simulink model "system_model_user_friendly"  (R2013a)
settings: Solver=ode15s  StartTime=0.0  StopTime=20  FixedStep=.00001  MaxStep=0.001  RelTol=1e-3
values from neighbouring files (symbols this model uses):
  Ga = 3    [a2_data_input_examsim1.m]    (also in a2_data_input_examsim2.m = 1; a2_data_input_hw3.m = 0.095; a2_data_input_mdcs_h5_v1_stud_p1.m = 0.095; a2_data_input_mdcs_h5_v1_stud_p4.m = 0.006)
  Gf = Gr/(Kd*Gs)    [a3_process_input.m]
  Gs = 1    [a2_data_input_examsim1.m]    (also in a2_data_input_examsim2.m = 5; a2_data_input_hw3.m; a2_data_input_mdcs_h5_v1_stud_p1.m; a2_data_input_mdcs_h5_v1_stud_p4.m)
  Kd = 2    [a2_data_input_examsim1.m]    (also in a2_data_input_examsim2.m = 1; a2_data_input_hw3.m = 1; a2_data_input_mdcs_h5_v1_stud_p1.m = 1; a2_data_input_mdcs_h5_v1_stud_p4.m = 1)
undefined symbols (not defined in the file or in its folder): da, dp, ds, r
libraries: cstblocks x2
settings Model: Creator=s177063  LastModifiedBy=Vittorio
settings DataIOCC: ExternalInput=[t,u]  LimitDataPoints=off  SaveOutput=off
settings OptimizationCC: ExpressionDepthLimit=2147483647
settings DebuggingCC: UnderspecifiedInitializationDetection=Simplified
settings GRTTargetCC: CombineOutputUpdateFcns=off  GRTInterface=on

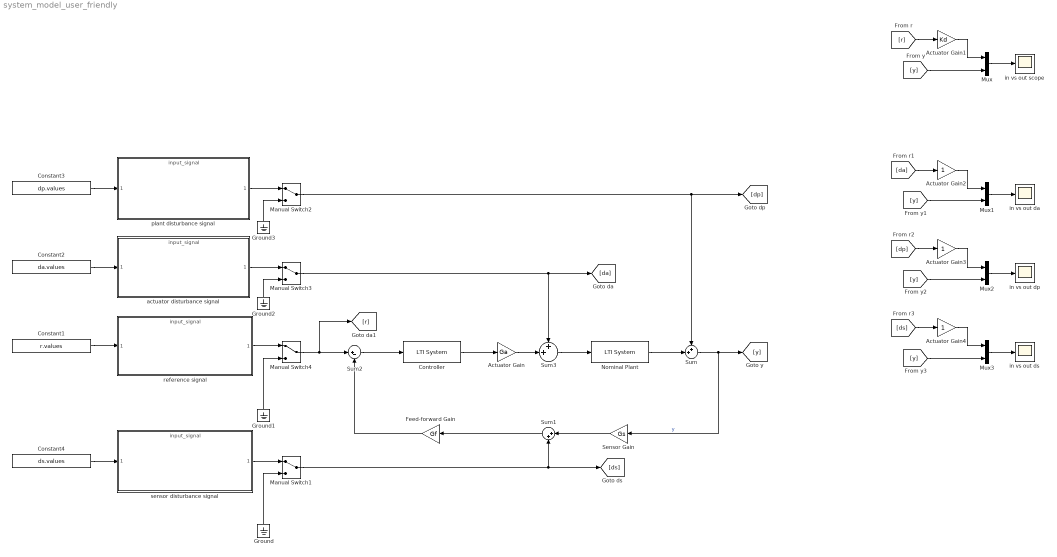
== system system_model_user_friendly ==
  Actuator Gain : Gain  Gain=Ga
  Actuator Gain1 : Gain  Gain=Kd
  Actuator Gain2 : Gain
  Actuator Gain3 : Gain
  Actuator Gain4 : Gain
  Constant1 : Constant  Value=r.values  OutDataTypeStr=Bus: slBus1
  Constant2 : Constant  Value=da.values  OutDataTypeStr=Bus: slBus1
  Constant3 : Constant  Value=dp.values  OutDataTypeStr=Bus: slBus1
  Constant4 : Constant  Value=ds.values  OutDataTypeStr=Bus: slBus1
  Controller : cstblocks/LTI System  sys=Gc.mod.value  IC=[]
  Feed-forward Gain : Gain  Gain=Gf
  Ground{,1..3} (4 alike) : Ground
  Manual Switch{1..4} (4 alike) : ManualSwitch
  Mux{,1..3} (4 alike) : Mux  Inputs=2
  Nominal Plant : cstblocks/LTI System  sys=Gp.nominal.tf  IC=[]
  Sensor Gain : Gain  Gain=Gs
  Sum : Sum  Inputs=++|
  Sum1 : Sum  Inputs=|++
  Sum2 : Sum  Inputs=|+-
  Sum3 : Sum  Inputs=++|
  actuator disturbance signal : ModelReference  ModelNameDialog=input_signal  ModelReferenceVersion=1.24  CopyOfModelName=input_signal  DefaultDataLogging=off
  in vs out da : Scope
      settings: TimeRange=0.5  YMin=0.00425  YMax=0.0085  SampleInput=on
  in vs out dp : Scope
      settings: TimeRange=0.5  YMin=7.45  YMax=8.3  SaveName=ScopeData2  SampleInput=on
  in vs out ds : Scope
      settings: TimeRange=0.5  YMin=-0.0012  YMax=0.0012  SaveName=ScopeData3  SampleInput=on
  in vs out scope : Scope
      settings: TimeRange=0.5  YMin=7.45  YMax=8.3  SampleInput=on
  plant disturbance signal : ModelReference  ModelNameDialog=input_signal  ModelReferenceVersion=1.24  CopyOfModelName=input_signal  DefaultDataLogging=off
  reference signal : ModelReference  ModelNameDialog=input_signal  ModelReferenceVersion=1.24  CopyOfModelName=input_signal  DefaultDataLogging=off
  sensor disturbance signal : ModelReference  ModelNameDialog=input_signal  ModelReferenceVersion=1.24  CopyOfModelName=input_signal  DefaultDataLogging=off
  wires:
  Sum/1 -> Sensor Gain/1, [y]  "y"
  Controller/1 -> Actuator Gain/1
  Sum3/1 -> Nominal Plant/1
  Sum2/1 -> Controller/1
  Sensor Gain/1 -> Sum1/1
  Sum1/1 -> Feed-forward Gain/1
  Feed-forward Gain/1 -> Sum2/2
  Actuator Gain/1 -> Sum3/2
  Nominal Plant/1 -> Sum/2
  Mux/1 -> in vs out scope/1
  [r] -> Actuator Gain1/1
  Actuator Gain1/1 -> Mux/1
  [y] -> Mux/2
  Constant1/1 -> reference signal/1
  Constant2/1 -> actuator disturbance signal/1
  Constant3/1 -> plant disturbance signal/1
  Constant4/1 -> sensor disturbance signal/1
  plant disturbance signal/1 -> Manual Switch2/1
  Manual Switch2/1 -> Sum/1, [dp]
  actuator disturbance signal/1 -> Manual Switch3/1
  reference signal/1 -> Manual Switch4/1
  Manual Switch4/1 -> [r], Sum2/1
  sensor disturbance signal/1 -> Manual Switch1/1
  Manual Switch1/1 -> Sum1/2, [ds]
  Ground/1 -> Manual Switch1/2
  Ground1/1 -> Manual Switch4/2
  Ground2/1 -> Manual Switch3/2
  Ground3/1 -> Manual Switch2/2
  Mux1/1 -> in vs out da/1
  [da] -> Actuator Gain2/1
  Actuator Gain2/1 -> Mux1/1
  [y] -> Mux1/2
  Mux2/1 -> in vs out dp/1
  [dp] -> Actuator Gain3/1
  Actuator Gain3/1 -> Mux2/1
  [y] -> Mux2/2
  Mux3/1 -> in vs out ds/1
  [ds] -> Actuator Gain4/1
  Actuator Gain4/1 -> Mux3/1
  [y] -> Mux3/2
  Manual Switch3/1 -> Sum3/1, [da]
